simulink library "Mixing_Valve"  (R2018b)
settings: Solver=ode45  StartTime=0.0  StopTime=10.0  RelTol=1e-3  EnableMultiTasking=on
undefined symbols (not defined in the file): linear
libraries: carnot x3, simulink x2
settings Model: Creator=lena.frank  LastModifiedBy=P41573
settings DataIOCC: LimitDataPoints=on  SaveFormat=Array  SignalLoggingSaveFormat=ModelDataLogs
settings OptimizationCC: ExpressionDepthLimit=2147483647  LifeSpan=inf
settings DebuggingCC: UnderspecifiedInitializationDetection=Classic  MergeDetectMultiDrivingBlocksExec=none  SolverPrmCheckMsg=warning  FcnCallInpInsideContextMsg=warning  StateNameClashWarn=warning  SFUnexpectedBacktrackingDiag=warning  SFNoUnconditionalDefaultTransitionDiag=warning  SFExecutionAtInitializationDiag=none
settings HardwareCC: ProdBitPerPointer=32  ProdBitPerSizeT=32  ProdBitPerPtrDiffT=32  ProdLargestAtomicFloat=None  ProdIntDivRoundTo=Undefined  ProdEndianess=Unspecified  ProdWordSize=32  ProdHWDeviceType=32-bit Generic
settings ModelReferenceCC: PropagateSignalLabelsOutOfModel=off
settings SFSimCC: SimUseLocalCustomCode=off
settings RTWCC: RTWUseLocalCustomCode=off
settings CodeAppCC: StateflowObjectComments=on
settings GRTTargetCC: TargetLangStandard=C89/C90 (ANSI)  GeneratePreprocessorConditionals=Disable all  CombineOutputUpdateFcns=off  GRTInterface=on
settings ConfigComp: CovMetricSettings=dw  CovHtmlReporting=on  CovSaveCumulativeToWorkspaceVar=on  CovSaveSingleToWorkspaceVar=on  CovExternalEMLEnable=off

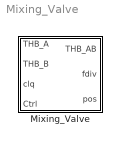
== system Mixing_Valve ==
  Mixing_Valve : Subsystem  mask(Mixing Valve){Art_A=equal percentage, Art_B=linear, kvs=1.6, psi_0=0.01, dt_V=30}
      mask prompts: Art_A "Valve characteristic A->AB"; Art_B "Valve characteristic B->AB"; kvs "Kvs: flow coefficient of the open valve in m³/h"; psi_0 "Psi_0: relative flow coefficient Kv/Kvs of the closed valve"; dt_V "Valve running time in s"
      mask help:
      | Mixes two massflows and calculates the pressure drop of the branches. The new temperature is calculated by an energy balance. The output f_div may be fed back to the corresponding flow diverter upwards in flowdirection.
      | This model uses a Memory block to break an algebraic loop. Avoid using the variable-step solver ode15s or ode113 (see block help for details).
      mask Help: web(fullfile(path_carnot('help'),'Mixing_Valve.html'),'-helpbrowser')
      mask TypeOptions Art_A: Valve_A/vtyp
      mask TypeOptions Art_B: Valve_B/vtyp
      mask TypeOptions kvs: Valve_A/kvs | Valve_B/kvs
      mask TypeOptions psi_0: Valve_A/psi_0 | Valve_B/psi_0
      mask TypeOptions dt_V: Valve_A/dt_V | Valve_B/dt_V
      mask Display:
      | plot(-20,-5,110,90,...
      |     [20 50 20 20],[20 30 40 20],...
      |     [50 80 80 50],[30 20 40 30],...
      |     [50 40 60 50],[30 10 10 30],...
      |     [50,50],[45,30],...
      |     [40,30,30,40,60,70,70,60,40],[45,50,60,65,65,60,50,45,45],...
      |     [60,60,50,40,40],[50,60,55,60,50])

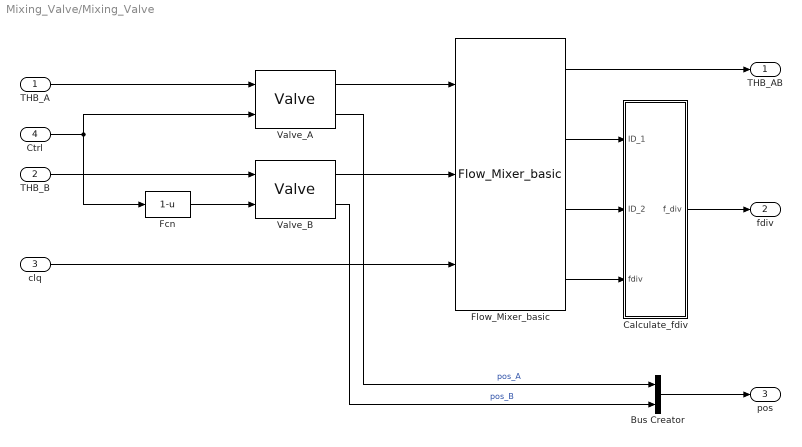
== system Mixing_Valve/Mixing_Valve ==
  THB_A : Inport
  THB_B : Inport  Port=2
  clq : Inport  Port=3
  Ctrl : Inport  Port=4
  Bus Creator : BusCreator  Inputs=2
  Calculate_fdiv : Subsystem
  Fcn : Fcn  Expr=1-u
  Flow_Mixer_basic : carnot/Basic/Hydraulics/Flow_Mixer_basic
      settings: SourceProductName=Carnot
  Valve_A : carnot/Hydraulics/Valve  vtyp=equal percentage  psi_0=psi_0  kvs=kvs  dt_V=dt_V
      settings: SourceProductName=Carnot
  Valve_B : carnot/Hydraulics/Valve  vtyp=linear  psi_0=psi_0  kvs=kvs  dt_V=dt_V
      settings: SourceProductName=Carnot
  THB_AB : Outport
  fdiv : Outport  Port=2
  pos : Outport  Port=3
  wires:
  Fcn/1 -> Valve_B/2
  Valve_B/2 -> Bus Creator/2  "pos_B"
  Valve_A/2 -> Bus Creator/1  "pos_A"
  Bus Creator/1 -> pos/1
  Valve_B/1 -> Flow_Mixer_basic/2
  Ctrl/1 -> Valve_A/2, Fcn/1
  THB_B/1 -> Valve_B/1
  Valve_A/1 -> Flow_Mixer_basic/1
  clq/1 -> Flow_Mixer_basic/3
  Calculate_fdiv/1(f_div) -> fdiv/1
  THB_A/1 -> Valve_A/1
  Flow_Mixer_basic/1 -> THB_AB/1
  Flow_Mixer_basic/2 -> Calculate_fdiv/1(ID_1)
  Flow_Mixer_basic/3 -> Calculate_fdiv/2(ID_2)
  Flow_Mixer_basic/4 -> Calculate_fdiv/3(fdiv)

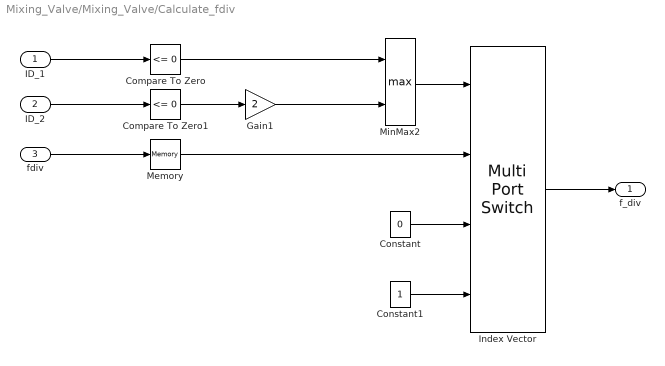
== system Mixing_Valve/Mixing_Valve/Calculate_fdiv ==
  ID_1 : Inport
  ID_2 : Inport  Port=2
  fdiv : Inport  Port=3
  Compare To Zero : simulink/Logic and Bit Operations/Compare To Zero  relop=<=  OutDataTypeStr=uint8
  Compare To Zero1 : simulink/Logic and Bit Operations/Compare To Zero  relop=<=  OutDataTypeStr=uint8
  Constant : Constant  Value=0
  Constant1 : Constant
  Gain1 : Gain  Gain=2
  Index Vector : MultiPortSwitch  DataPortOrder=Zero-based contiguous  zeroidx=on
  Memory : Memory
  MinMax2 : MinMax  Function=max  Inputs=2
  f_div : Outport
  wires:
  Memory/1 -> Index Vector/2
  Compare To Zero1/1 -> Gain1/1
  Compare To Zero/1 -> MinMax2/1
  MinMax2/1 -> Index Vector/1
  ID_1/1 -> Compare To Zero/1
  ID_2/1 -> Compare To Zero1/1
  Constant/1 -> Index Vector/3
  fdiv/1 -> Memory/1
  Constant1/1 -> Index Vector/4
  Gain1/1 -> MinMax2/2
  Index Vector/1 -> f_div/1
